simulink model "Distribution_v2"  (Simulink 7.9)
settings: Solver=VariableStepDiscrete  StartTime=0.0  StopTime=1000  RelTol=1e-3
libraries: simeventslib x35
(part 1 of 6)
settings Model: Creator=tsprock3  LastModifiedBy=tsprock3
settings DebuggingCC: SimStateOlderReleaseMsg=warning

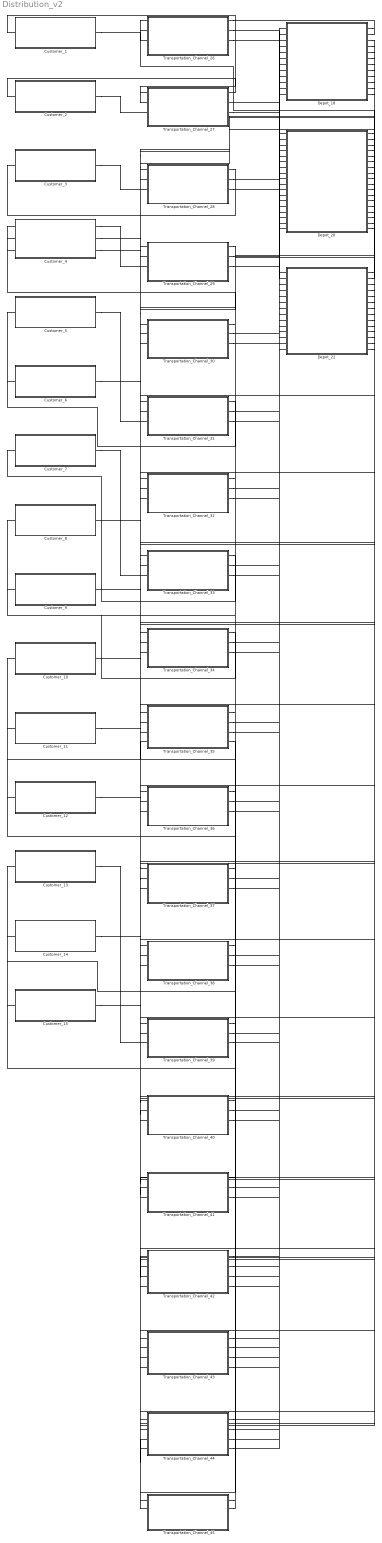
== system Distribution_v2 ==
  Customer_1 : Subsystem
  Customer_10 : Subsystem
  Customer_11 : Subsystem
  Customer_12 : Subsystem
  Customer_13 : Subsystem
  Customer_14 : Subsystem
  Customer_15 : Subsystem
  Customer_2 : Subsystem
  Customer_3 : Subsystem
  Customer_4 : Subsystem
  Customer_5 : Subsystem
  Customer_6 : Subsystem
  Customer_7 : Subsystem
  Customer_8 : Subsystem
  Customer_9 : Subsystem
  Depot_18 : Subsystem
  Depot_20 : Subsystem
  Depot_22 : Subsystem
  Transportation_Channel_26 : Subsystem
  Transportation_Channel_27 : Subsystem
  Transportation_Channel_28 : Subsystem
  Transportation_Channel_29 : Subsystem
  Transportation_Channel_30 : Subsystem
  Transportation_Channel_31 : Subsystem
  Transportation_Channel_32 : Subsystem
  Transportation_Channel_33 : Subsystem
  Transportation_Channel_34 : Subsystem
  Transportation_Channel_35 : Subsystem
  Transportation_Channel_36 : Subsystem
  Transportation_Channel_37 : Subsystem
  Transportation_Channel_38 : Subsystem
  Transportation_Channel_39 : Subsystem
  Transportation_Channel_40 : Subsystem
  Transportation_Channel_41 : Subsystem
  Transportation_Channel_42 : Subsystem
  Transportation_Channel_43 : Subsystem
  Transportation_Channel_44 : Subsystem
  Transportation_Channel_45 : Subsystem
  connections:
  Depot_22/RConn1 -- Transportation_Channel_26/LConn1
  Transportation_Channel_26/RConn1 -- Customer_1/LConn1
  Depot_22/RConn2 -- Transportation_Channel_26/LConn2
  Transportation_Channel_26/RConn2 -- Depot_22/LConn1
  Customer_1/RConn1 -- Transportation_Channel_26/LConn3
  Transportation_Channel_26/RConn3 -- Depot_22/LConn2
  Depot_18/RConn1 -- Transportation_Channel_27/LConn1
  Transportation_Channel_27/RConn1 -- Customer_2/LConn1
  Depot_18/RConn2 -- Transportation_Channel_27/LConn2
  Transportation_Channel_27/RConn2 -- Depot_18/LConn1
  Customer_2/RConn1 -- Transportation_Channel_27/LConn3
  Transportation_Channel_27/RConn3 -- Depot_18/LConn2
  Depot_20/RConn1 -- Transportation_Channel_28/LConn1
  Transportation_Channel_28/RConn1 -- Customer_3/LConn1
  Depot_20/RConn2 -- Transportation_Channel_28/LConn2
  Transportation_Channel_28/RConn2 -- Depot_20/LConn1
  Customer_3/RConn1 -- Transportation_Channel_28/LConn3
  Transportation_Channel_28/RConn3 -- Depot_20/LConn2
  Depot_18/RConn3 -- Transportation_Channel_29/LConn1
  Transportation_Channel_29/RConn1 -- Customer_4/LConn1
  Depot_18/RConn4 -- Transportation_Channel_29/LConn2
  Transportation_Channel_29/RConn2 -- Depot_18/LConn3
  Customer_4/RConn1 -- Transportation_Channel_29/LConn3
  Transportation_Channel_29/RConn3 -- Depot_18/LConn4
  Depot_20/RConn3 -- Transportation_Channel_30/LConn1
  Transportation_Channel_30/RConn1 -- Customer_4/LConn2
  Depot_20/RConn4 -- Transportation_Channel_30/LConn2
  Transportation_Channel_30/RConn2 -- Depot_20/LConn3
  Customer_4/RConn2 -- Transportation_Channel_30/LConn3
  Transportation_Channel_30/RConn3 -- Depot_20/LConn4
  Depot_22/RConn3 -- Transportation_Channel_31/LConn1
  Transportation_Channel_31/RConn1 -- Customer_5/LConn1
  Depot_22/RConn4 -- Transportation_Channel_31/LConn2
  Transportation_Channel_31/RConn2 -- Depot_22/LConn3
  Customer_5/RConn1 -- Transportation_Channel_31/LConn3
  Transportation_Channel_31/RConn3 -- Depot_22/LConn4
  Depot_18/RConn5 -- Transportation_Channel_32/LConn1
  Transportation_Channel_32/RConn1 -- Customer_6/LConn1
  Depot_18/RConn6 -- Transportation_Channel_32/LConn2
  Transportation_Channel_32/RConn2 -- Depot_18/LConn5
  Customer_6/RConn1 -- Transportation_Channel_32/LConn3
  Transportation_Channel_32/RConn3 -- Depot_18/LConn6
  Depot_20/RConn5 -- Transportation_Channel_33/LConn1
  Transportation_Channel_33/RConn1 -- Customer_7/LConn1
  Depot_20/RConn6 -- Transportation_Channel_33/LConn2
  Transportation_Channel_33/RConn2 -- Depot_20/LConn5
  Customer_7/RConn1 -- Transportation_Channel_33/LConn3
  Transportation_Channel_33/RConn3 -- Depot_20/LConn6
  Depot_20/RConn7 -- Transportation_Channel_34/LConn1
  Transportation_Channel_34/RConn1 -- Customer_8/LConn1
  Depot_20/RConn8 -- Transportation_Channel_34/LConn2
  Transportation_Channel_34/RConn2 -- Depot_20/LConn7
  Customer_8/RConn1 -- Transportation_Channel_34/LConn3
  Transportation_Channel_34/RConn3 -- Depot_20/LConn8
  Depot_18/RConn7 -- Transportation_Channel_35/LConn1
  Transportation_Channel_35/RConn1 -- Customer_9/LConn1
  Depot_18/RConn8 -- Transportation_Channel_35/LConn2
  Transportation_Channel_35/RConn2 -- Depot_18/LConn7
  Customer_9/RConn1 -- Transportation_Channel_35/LConn3
  Transportation_Channel_35/RConn3 -- Depot_18/LConn8
  Depot_22/RConn5 -- Transportation_Channel_36/LConn1
  Transportation_Channel_36/RConn1 -- Customer_10/LConn1
  Depot_22/RConn6 -- Transportation_Channel_36/LConn2
  Transportation_Channel_36/RConn2 -- Depot_22/LConn5
  Customer_10/RConn1 -- Transportation_Channel_36/LConn3
  Transportation_Channel_36/RConn3 -- Depot_22/LConn6
  Depot_20/RConn9 -- Transportation_Channel_37/LConn1
  Transportation_Channel_37/RConn1 -- Customer_11/LConn1
  Depot_20/RConn10 -- Transportation_Channel_37/LConn2
  Transportation_Channel_37/RConn2 -- Depot_20/LConn9
  Customer_11/RConn1 -- Transportation_Channel_37/LConn3
  Transportation_Channel_37/RConn3 -- Depot_20/LConn10
  Depot_22/RConn7 -- Transportation_Channel_38/LConn1
  Transportation_Channel_38/RConn1 -- Customer_12/LConn1
  Depot_22/RConn8 -- Transportation_Channel_38/LConn2
  Transportation_Channel_38/RConn2 -- Depot_22/LConn7
  Customer_12/RConn1 -- Transportation_Channel_38/LConn3
  Transportation_Channel_38/RConn3 -- Depot_22/LConn8
  Depot_22/RConn9 -- Transportation_Channel_39/LConn1
  Transportation_Channel_39/RConn1 -- Customer_13/LConn1
  Depot_22/RConn10 -- Transportation_Channel_39/LConn2
  Transportation_Channel_39/RConn2 -- Depot_22/LConn9
  Customer_13/RConn1 -- Transportation_Channel_39/LConn3
  Transportation_Channel_39/RConn3 -- Depot_22/LConn10
  Depot_20/RConn11 -- Transportation_Channel_40/LConn1
  Transportation_Channel_40/RConn1 -- Customer_14/LConn1
  Depot_20/RConn12 -- Transportation_Channel_40/LConn2
  Transportation_Channel_40/RConn2 -- Depot_20/LConn11
  Customer_14/RConn1 -- Transportation_Channel_40/LConn3
  Transportation_Channel_40/RConn3 -- Depot_20/LConn12
  Depot_20/RConn13 -- Transportation_Channel_41/LConn1
  Transportation_Channel_41/RConn1 -- Customer_15/LConn1
  Depot_20/RConn14 -- Transportation_Channel_41/LConn2
  Transportation_Channel_41/RConn2 -- Depot_20/LConn13
  Customer_15/RConn1 -- Transportation_Channel_41/LConn3
  Transportation_Channel_41/RConn3 -- Depot_20/LConn14
  Depot_20/RConn15 -- Transportation_Channel_42/LConn1
  Transportation_Channel_42/RConn1 -- Depot_18/LConn9
  Depot_20/RConn16 -- Transportation_Channel_42/LConn2
  Transportation_Channel_42/RConn2 -- Depot_20/LConn15
  Depot_18/RConn9 -- Transportation_Channel_42/LConn3
  Transportation_Channel_42/RConn3 -- Depot_20/LConn16
  Depot_18/RConn10 -- Transportation_Channel_42/LConn4
  Transportation_Channel_42/RConn4 -- Depot_18/LConn10
  Depot_22/RConn11 -- Transportation_Channel_43/LConn1
  Transportation_Channel_43/RConn1 -- Depot_18/LConn11
  Depot_22/RConn12 -- Transportation_Channel_43/LConn2
  Transportation_Channel_43/RConn2 -- Depot_22/LConn11
  Depot_18/RConn11 -- Transportation_Channel_43/LConn3
  Transportation_Channel_43/RConn3 -- Depot_22/LConn12
  Depot_18/RConn12 -- Transportation_Channel_43/LConn4
  Transportation_Channel_43/RConn4 -- Depot_18/LConn12
  Depot_22/RConn13 -- Transportation_Channel_44/LConn1
  Transportation_Channel_44/RConn1 -- Depot_20/LConn17
  Depot_22/RConn14 -- Transportation_Channel_44/LConn2
  Transportation_Channel_44/RConn2 -- Depot_22/LConn13
  Depot_20/RConn17 -- Transportation_Channel_44/LConn3
  Transportation_Channel_44/RConn3 -- Depot_22/LConn14
  Depot_20/RConn18 -- Transportation_Channel_44/LConn4
  Transportation_Channel_44/RConn4 -- Depot_20/LConn18
  Transportation_Channel_35/RConn4 -- Transportation_Channel_45/LConn1
  Transportation_Channel_45/RConn1 -- Customer_4/LConn3
  Customer_4/RConn3 -- Transportation_Channel_45/LConn2
  Transportation_Channel_45/RConn2 -- Transportation_Channel_35/LConn4

== system Distribution_v2/Customer_1 ==
  Commodity_1 : Subsystem  mask{Mean=2000/340, AttributeValue=[1  22  18   2]|1|2|1}
      mask prompts: Mean "Frequency"; AttributeValue "Attributes"
  Commodity_2 : Subsystem  mask{Mean=2000/60, AttributeValue=[1  22  18   4]|1|4|1}
      mask prompts: Mean "Frequency"; AttributeValue "Attributes"
  Commodity_3 : Subsystem  mask{Mean=2000/480, AttributeValue=[1  22   5   0]|1|5|1}
      mask prompts: Mean "Frequency"; AttributeValue "Attributes"
  Commodity_4 : Subsystem  mask{Mean=2000/293, AttributeValue=[1  22  18   6]|1|6|1}
      mask prompts: Mean "Frequency"; AttributeValue "Attributes"
  Commodity_5 : Subsystem  mask{Mean=2000/376, AttributeValue=[1  22  20   7]|1|7|1}
      mask prompts: Mean "Frequency"; AttributeValue "Attributes"
  Commodity_6 : Subsystem  mask{Mean=2000/253, AttributeValue=[1  22  20   8]|1|8|1}
      mask prompts: Mean "Frequency"; AttributeValue "Attributes"
  Commodity_7 : Subsystem  mask{Mean=2000/75, AttributeValue=[1  22  13   0]|1|13|1}
      mask prompts: Mean "Frequency"; AttributeValue "Attributes"
  Commodity_8 : Subsystem  mask{Mean=2000/421, AttributeValue=[1  22  20  14]|1|14|1}
      mask prompts: Mean "Frequency"; AttributeValue "Attributes"
  Commodity_9 : Subsystem  mask{Mean=2000/408, AttributeValue=[1  22  20  15]|1|15|1}
      mask prompts: Mean "Frequency"; AttributeValue "Attributes"
  Entity Sink : EntitySink
  Get Attribute : GetAttribute  AttributeName=Origin|Destination|Start  AttributeMissing=Error|Error|Error  AttributeDefaultValue=1|1|1  AttributeTreatAsVector=1|1|1  AttributeSendTiming=After entity departure|After entity departure|After entity departure  EvaluatedDefaultAttributeValue={[];[];[]}
      settings: OutputPortMap=o1,o2,o3
  Get Attribute1 : GetAttribute  AttributeName=Route  EvaluatedDefaultAttributeValue={[]}
      settings: OutputPortMap=o1
  IN_Commodity : PathCombiner  NumberInputPorts=9
  IN_Shipment : PathCombiner  NumberInputPorts=1
  Lookup : Constant  Value=[22]
  MATLAB Function : MATLAB Function  TreatAsAtomicUnit=on
  Mux : Mux  Inputs=3
  Node_ID : Constant
  OUT_Shipment : OutputSwitch  NumberOutputPorts=1  SwitchingCriterion=From signal port p  AttributeName=Customer
  Shipment_Metrics : simeventslib/SimEvents Sinks/Discrete Event Signal to Workspace  VariableName=Customer_1  SaveFormat=Structure With Time  isMonitorOnly=off  isRecordIC=off
  Single Server : SingleServer  ServiceTime=0
  Timed to Evnt Signal : TimedToEventSignal
  Timed to Evnt Signal1 : TimedToEventSignal
  IN_Shipment_1 : PMIOPort  Port=1  Side=Left
  OUT_Shipment_1 : PMIOPort  Port=2  Side=Right
  wires:
  Timed to Evnt Signal1/1 -> MATLAB Function/3(lookup)
  Lookup/1 -> Timed to Evnt Signal1/1
  Timed to Evnt Signal/1 -> MATLAB Function/2(current)
  Get Attribute1/1 -> MATLAB Function/1(route)
  MATLAB Function/1(next) -> OUT_Shipment/1
  Node_ID/1 -> Timed to Evnt Signal/1
  Mux/1 -> Shipment_Metrics/1
  Get Attribute/3 -> Mux/3
  Get Attribute/2 -> Mux/2
  Get Attribute/1 -> Mux/1
  connections:
  Single Server/RConn1 -- OUT_Shipment/LConn1
  Get Attribute1/RConn1 -- Single Server/LConn1
  IN_Commodity/RConn1 -- Get Attribute1/LConn1
  Get Attribute/LConn1 -- IN_Shipment/RConn1
  Entity Sink/LConn1 -- Get Attribute/RConn1
  IN_Shipment/LConn1 -- IN_Shipment_1/RConn1
  OUT_Shipment/RConn1 -- OUT_Shipment_1/RConn1
  Commodity_1/RConn1 -- IN_Commodity/LConn1
  Commodity_2/RConn1 -- IN_Commodity/LConn2
  Commodity_3/RConn1 -- IN_Commodity/LConn3
  Commodity_4/RConn1 -- IN_Commodity/LConn4
  Commodity_5/RConn1 -- IN_Commodity/LConn5
  Commodity_6/RConn1 -- IN_Commodity/LConn6
  Commodity_7/RConn1 -- IN_Commodity/LConn7
  Commodity_8/RConn1 -- IN_Commodity/LConn8
  Commodity_9/RConn1 -- IN_Commodity/LConn9

== system Distribution_v2/Customer_10 ==
  Commodity_75 : Subsystem  mask{Mean=2000/245, AttributeValue=[10  22  18   4]|10|4|1}
      mask prompts: Mean "Frequency"; AttributeValue "Attributes"
  Commodity_76 : Subsystem  mask{Mean=2000/184, AttributeValue=[10  22  20   7]|10|7|1}
      mask prompts: Mean "Frequency"; AttributeValue "Attributes"
  Commodity_77 : Subsystem  mask{Mean=2000/443, AttributeValue=[10  22  18   9]|10|9|1}
      mask prompts: Mean "Frequency"; AttributeValue "Attributes"
  Commodity_78 : Subsystem  mask{Mean=2000/131, AttributeValue=[10  22  13   0]|10|13|1}
      mask prompts: Mean "Frequency"; AttributeValue "Attributes"
  Commodity_79 : Subsystem  mask{Mean=2000/340, AttributeValue=[10  22  20  14]|10|14|1}
      mask prompts: Mean "Frequency"; AttributeValue "Attributes"
  Commodity_80 : Subsystem  mask{Mean=2000/361, AttributeValue=[10  22  20  15]|10|15|1}
      mask prompts: Mean "Frequency"; AttributeValue "Attributes"
  Entity Sink : EntitySink
  Get Attribute : GetAttribute  AttributeName=Origin|Destination|Start  AttributeMissing=Error|Error|Error  AttributeDefaultValue=1|1|1  AttributeTreatAsVector=1|1|1  AttributeSendTiming=After entity departure|After entity departure|After entity departure  EvaluatedDefaultAttributeValue={[];[];[]}
      settings: OutputPortMap=o1,o2,o3
  Get Attribute1 : GetAttribute  AttributeName=Route  EvaluatedDefaultAttributeValue={[]}
      settings: OutputPortMap=o1
  IN_Commodity : PathCombiner  NumberInputPorts=6
  IN_Shipment : PathCombiner  NumberInputPorts=1
  Lookup : Constant  Value=[22]
  MATLAB Function : MATLAB Function  TreatAsAtomicUnit=on
  Mux : Mux  Inputs=3
  Node_ID : Constant  Value=10
  OUT_Shipment : OutputSwitch  NumberOutputPorts=1  SwitchingCriterion=From signal port p  AttributeName=Customer
  Shipment_Metrics : simeventslib/SimEvents Sinks/Discrete Event Signal to Workspace  VariableName=Customer_10  SaveFormat=Structure With Time  isMonitorOnly=off  isRecordIC=off
  Single Server : SingleServer  ServiceTime=0
  Timed to Evnt Signal : TimedToEventSignal
  Timed to Evnt Signal1 : TimedToEventSignal
  IN_Shipment_1 : PMIOPort  Port=1  Side=Left
  OUT_Shipment_1 : PMIOPort  Port=2  Side=Right
  wires:
  Timed to Evnt Signal1/1 -> MATLAB Function/3(lookup)
  Lookup/1 -> Timed to Evnt Signal1/1
  Timed to Evnt Signal/1 -> MATLAB Function/2(current)
  Get Attribute1/1 -> MATLAB Function/1(route)
  MATLAB Function/1(next) -> OUT_Shipment/1
  Node_ID/1 -> Timed to Evnt Signal/1
  Mux/1 -> Shipment_Metrics/1
  Get Attribute/3 -> Mux/3
  Get Attribute/2 -> Mux/2
  Get Attribute/1 -> Mux/1
  connections:
  Single Server/RConn1 -- OUT_Shipment/LConn1
  Get Attribute1/RConn1 -- Single Server/LConn1
  IN_Commodity/RConn1 -- Get Attribute1/LConn1
  Get Attribute/LConn1 -- IN_Shipment/RConn1
  Entity Sink/LConn1 -- Get Attribute/RConn1
  IN_Shipment/LConn1 -- IN_Shipment_1/RConn1
  OUT_Shipment/RConn1 -- OUT_Shipment_1/RConn1
  Commodity_75/RConn1 -- IN_Commodity/LConn1
  Commodity_76/RConn1 -- IN_Commodity/LConn2
  Commodity_77/RConn1 -- IN_Commodity/LConn3
  Commodity_78/RConn1 -- IN_Commodity/LConn4
  Commodity_79/RConn1 -- IN_Commodity/LConn5
  Commodity_80/RConn1 -- IN_Commodity/LConn6

== system Distribution_v2/Customer_11 ==
  Commodity_81 : Subsystem  mask{Mean=2000/327, AttributeValue=[11  20  22   1]|11|1|1}
      mask prompts: Mean "Frequency"; AttributeValue "Attributes"
  Commodity_82 : Subsystem  mask{Mean=2000/390, AttributeValue=[11  20  18   2]|11|2|1}
      mask prompts: Mean "Frequency"; AttributeValue "Attributes"
  Commodity_83 : Subsystem  mask{Mean=2000/350, AttributeValue=[11  20  18   6]|11|6|1}
      mask prompts: Mean "Frequency"; AttributeValue "Attributes"
  Commodity_84 : Subsystem  mask{Mean=2000/16, AttributeValue=[11  20   7   0]|11|7|1}
      mask prompts: Mean "Frequency"; AttributeValue "Attributes"
  Commodity_85 : Subsystem  mask{Mean=2000/453, AttributeValue=[11  20  22  10]|11|10|1}
      mask prompts: Mean "Frequency"; AttributeValue "Attributes"
  Entity Sink : EntitySink
  Get Attribute : GetAttribute  AttributeName=Origin|Destination|Start  AttributeMissing=Error|Error|Error  AttributeDefaultValue=1|1|1  AttributeTreatAsVector=1|1|1  AttributeSendTiming=After entity departure|After entity departure|After entity departure  EvaluatedDefaultAttributeValue={[];[];[]}
      settings: OutputPortMap=o1,o2,o3
  Get Attribute1 : GetAttribute  AttributeName=Route  EvaluatedDefaultAttributeValue={[]}
      settings: OutputPortMap=o1
  IN_Commodity : PathCombiner  NumberInputPorts=5
  IN_Shipment : PathCombiner  NumberInputPorts=1
  Lookup : Constant  Value=[20]
  MATLAB Function : MATLAB Function  TreatAsAtomicUnit=on
  Mux : Mux  Inputs=3
  Node_ID : Constant  Value=11
  OUT_Shipment : OutputSwitch  NumberOutputPorts=1  SwitchingCriterion=From signal port p  AttributeName=Customer
  Shipment_Metrics : simeventslib/SimEvents Sinks/Discrete Event Signal to Workspace  VariableName=Customer_11  SaveFormat=Structure With Time  isMonitorOnly=off  isRecordIC=off
  Single Server : SingleServer  ServiceTime=0
  Timed to Evnt Signal : TimedToEventSignal
  Timed to Evnt Signal1 : TimedToEventSignal
  IN_Shipment_1 : PMIOPort  Port=1  Side=Left
  OUT_Shipment_1 : PMIOPort  Port=2  Side=Right
  wires:
  Timed to Evnt Signal1/1 -> MATLAB Function/3(lookup)
  Lookup/1 -> Timed to Evnt Signal1/1
  Timed to Evnt Signal/1 -> MATLAB Function/2(current)
  Get Attribute1/1 -> MATLAB Function/1(route)
  MATLAB Function/1(next) -> OUT_Shipment/1
  Node_ID/1 -> Timed to Evnt Signal/1
  Mux/1 -> Shipment_Metrics/1
  Get Attribute/3 -> Mux/3
  Get Attribute/2 -> Mux/2
  Get Attribute/1 -> Mux/1
  connections:
  Single Server/RConn1 -- OUT_Shipment/LConn1
  Get Attribute1/RConn1 -- Single Server/LConn1
  IN_Commodity/RConn1 -- Get Attribute1/LConn1
  Get Attribute/LConn1 -- IN_Shipment/RConn1
  Entity Sink/LConn1 -- Get Attribute/RConn1
  IN_Shipment/LConn1 -- IN_Shipment_1/RConn1
  OUT_Shipment/RConn1 -- OUT_Shipment_1/RConn1
  Commodity_81/RConn1 -- IN_Commodity/LConn1
  Commodity_82/RConn1 -- IN_Commodity/LConn2
  Commodity_83/RConn1 -- IN_Commodity/LConn3
  Commodity_84/RConn1 -- IN_Commodity/LConn4
  Commodity_85/RConn1 -- IN_Commodity/LConn5

== system Distribution_v2/Customer_12 ==
  Commodity_86 : Subsystem  mask{Mean=2000/120, AttributeValue=[12  22  18   2]|12|2|1}
      mask prompts: Mean "Frequency"; AttributeValue "Attributes"
  Commodity_87 : Subsystem  mask{Mean=2000/245, AttributeValue=[12  22  18   4]|12|4|1}
      mask prompts: Mean "Frequency"; AttributeValue "Attributes"
  Commodity_88 : Subsystem  mask{Mean=2000/490, AttributeValue=[12  22   5   0]|12|5|1}
      mask prompts: Mean "Frequency"; AttributeValue "Attributes"
  Commodity_89 : Subsystem  mask{Mean=2000/30, AttributeValue=[12  22  20   8]|12|8|1}
      mask prompts: Mean "Frequency"; AttributeValue "Attributes"
  Commodity_90 : Subsystem  mask{Mean=2000/36, AttributeValue=[12  22  10   0]|12|10|1}
      mask prompts: Mean "Frequency"; AttributeValue "Attributes"
  Commodity_91 : Subsystem  mask{Mean=2000/410, AttributeValue=[12  22  13   0]|12|13|1}
      mask prompts: Mean "Frequency"; AttributeValue "Attributes"
  Entity Sink : EntitySink
  Get Attribute : GetAttribute  AttributeName=Origin|Destination|Start  AttributeMissing=Error|Error|Error  AttributeDefaultValue=1|1|1  AttributeTreatAsVector=1|1|1  AttributeSendTiming=After entity departure|After entity departure|After entity departure  EvaluatedDefaultAttributeValue={[];[];[]}
      settings: OutputPortMap=o1,o2,o3
  Get Attribute1 : GetAttribute  AttributeName=Route  EvaluatedDefaultAttributeValue={[]}
      settings: OutputPortMap=o1
  IN_Commodity : PathCombiner  NumberInputPorts=6
  IN_Shipment : PathCombiner  NumberInputPorts=1
  Lookup : Constant  Value=[22]
  MATLAB Function : MATLAB Function  TreatAsAtomicUnit=on
  Mux : Mux  Inputs=3
  Node_ID : Constant  Value=12
  OUT_Shipment : OutputSwitch  NumberOutputPorts=1  SwitchingCriterion=From signal port p  AttributeName=Customer
  Shipment_Metrics : simeventslib/SimEvents Sinks/Discrete Event Signal to Workspace  VariableName=Customer_12  SaveFormat=Structure With Time  isMonitorOnly=off  isRecordIC=off
  Single Server : SingleServer  ServiceTime=0
  Timed to Evnt Signal : TimedToEventSignal
  Timed to Evnt Signal1 : TimedToEventSignal
  IN_Shipment_1 : PMIOPort  Port=1  Side=Left
  OUT_Shipment_1 : PMIOPort  Port=2  Side=Right
  wires:
  Timed to Evnt Signal1/1 -> MATLAB Function/3(lookup)
  Lookup/1 -> Timed to Evnt Signal1/1
  Timed to Evnt Signal/1 -> MATLAB Function/2(current)
  Get Attribute1/1 -> MATLAB Function/1(route)
  MATLAB Function/1(next) -> OUT_Shipment/1
  Node_ID/1 -> Timed to Evnt Signal/1
  Mux/1 -> Shipment_Metrics/1
  Get Attribute/3 -> Mux/3
  Get Attribute/2 -> Mux/2
  Get Attribute/1 -> Mux/1
  connections:
  Single Server/RConn1 -- OUT_Shipment/LConn1
  Get Attribute1/RConn1 -- Single Server/LConn1
  IN_Commodity/RConn1 -- Get Attribute1/LConn1
  Get Attribute/LConn1 -- IN_Shipment/RConn1
  Entity Sink/LConn1 -- Get Attribute/RConn1
  IN_Shipment/LConn1 -- IN_Shipment_1/RConn1
  OUT_Shipment/RConn1 -- OUT_Shipment_1/RConn1
  Commodity_86/RConn1 -- IN_Commodity/LConn1
  Commodity_87/RConn1 -- IN_Commodity/LConn2
  Commodity_88/RConn1 -- IN_Commodity/LConn3
  Commodity_89/RConn1 -- IN_Commodity/LConn4
  Commodity_90/RConn1 -- IN_Commodity/LConn5
  Commodity_91/RConn1 -- IN_Commodity/LConn6

== system Distribution_v2/Customer_13 ==
  Commodity_92 : Subsystem  mask{Mean=2000/330, AttributeValue=[13  22   1   0]|13|1|1}
      mask prompts: Mean "Frequency"; AttributeValue "Attributes"
  Commodity_93 : Subsystem  mask{Mean=2000/217, AttributeValue=[13  22  18   6]|13|6|1}
      mask prompts: Mean "Frequency"; AttributeValue "Attributes"
  Commodity_94 : Subsystem  mask{Mean=2000/67, AttributeValue=[13  22  20   8]|13|8|1}
      mask prompts: Mean "Frequency"; AttributeValue "Attributes"
  Commodity_95 : Subsystem  mask{Mean=2000/196, AttributeValue=[13  22  18   9]|13|9|1}
      mask prompts: Mean "Frequency"; AttributeValue "Attributes"
  Commodity_96 : Subsystem  mask{Mean=2000/200, AttributeValue=[13  22  12   0]|13|12|1}
      mask prompts: Mean "Frequency"; AttributeValue "Attributes"
  Commodity_97 : Subsystem  mask{Mean=2000/329, AttributeValue=[13  22  20  15]|13|15|1}
      mask prompts: Mean "Frequency"; AttributeValue "Attributes"
  Entity Sink : EntitySink
  Get Attribute : GetAttribute  AttributeName=Origin|Destination|Start  AttributeMissing=Error|Error|Error  AttributeDefaultValue=1|1|1  AttributeTreatAsVector=1|1|1  AttributeSendTiming=After entity departure|After entity departure|After entity departure  EvaluatedDefaultAttributeValue={[];[];[]}
      settings: OutputPortMap=o1,o2,o3
  Get Attribute1 : GetAttribute  AttributeName=Route  EvaluatedDefaultAttributeValue={[]}
      settings: OutputPortMap=o1
  IN_Commodity : PathCombiner  NumberInputPorts=6
  IN_Shipment : PathCombiner  NumberInputPorts=1
  Lookup : Constant  Value=[22]
  MATLAB Function : MATLAB Function  TreatAsAtomicUnit=on
  Mux : Mux  Inputs=3
  Node_ID : Constant  Value=13
  OUT_Shipment : OutputSwitch  NumberOutputPorts=1  SwitchingCriterion=From signal port p  AttributeName=Customer
  Shipment_Metrics : simeventslib/SimEvents Sinks/Discrete Event Signal to Workspace  VariableName=Customer_13  SaveFormat=Structure With Time  isMonitorOnly=off  isRecordIC=off
  Single Server : SingleServer  ServiceTime=0
  Timed to Evnt Signal : TimedToEventSignal
  Timed to Evnt Signal1 : TimedToEventSignal
  IN_Shipment_1 : PMIOPort  Port=1  Side=Left
  OUT_Shipment_1 : PMIOPort  Port=2  Side=Right
  wires:
  Timed to Evnt Signal1/1 -> MATLAB Function/3(lookup)
  Lookup/1 -> Timed to Evnt Signal1/1
  Timed to Evnt Signal/1 -> MATLAB Function/2(current)
  Get Attribute1/1 -> MATLAB Function/1(route)
  MATLAB Function/1(next) -> OUT_Shipment/1
  Node_ID/1 -> Timed to Evnt Signal/1
  Mux/1 -> Shipment_Metrics/1
  Get Attribute/3 -> Mux/3
  Get Attribute/2 -> Mux/2
  Get Attribute/1 -> Mux/1
  connections:
  Single Server/RConn1 -- OUT_Shipment/LConn1
  Get Attribute1/RConn1 -- Single Server/LConn1
  IN_Commodity/RConn1 -- Get Attribute1/LConn1
  Get Attribute/LConn1 -- IN_Shipment/RConn1
  Entity Sink/LConn1 -- Get Attribute/RConn1
  IN_Shipment/LConn1 -- IN_Shipment_1/RConn1
  OUT_Shipment/RConn1 -- OUT_Shipment_1/RConn1
  Commodity_92/RConn1 -- IN_Commodity/LConn1
  Commodity_93/RConn1 -- IN_Commodity/LConn2
  Commodity_94/RConn1 -- IN_Commodity/LConn3
  Commodity_95/RConn1 -- IN_Commodity/LConn4
  Commodity_96/RConn1 -- IN_Commodity/LConn5
  Commodity_97/RConn1 -- IN_Commodity/LConn6

== system Distribution_v2/Customer_14 ==
  Commodity_100 : Subsystem  mask{Mean=2000/54, AttributeValue=[14  20  18   4]|14|4|1}
      mask prompts: Mean "Frequency"; AttributeValue "Attributes"
  Commodity_101 : Subsystem  mask{Mean=2000/100, AttributeValue=[14  20  22   5]|14|5|1}
      mask prompts: Mean "Frequency"; AttributeValue "Attributes"
  Commodity_102 : Subsystem  mask{Mean=2000/170, AttributeValue=[14  20  18   6]|14|6|1}
      mask prompts: Mean "Frequency"; AttributeValue "Attributes"
  Commodity_103 : Subsystem  mask{Mean=2000/369, AttributeValue=[14  20  18   9]|14|9|1}
      mask prompts: Mean "Frequency"; AttributeValue "Attributes"
  Commodity_104 : Subsystem  mask{Mean=2000/212, AttributeValue=[14  20  22  10]|14|10|1}
      mask prompts: Mean "Frequency"; AttributeValue "Attributes"
  Commodity_105 : Subsystem  mask{Mean=2000/492, AttributeValue=[14  20  22  13]|14|13|1}
      mask prompts: Mean "Frequency"; AttributeValue "Attributes"
  Commodity_106 : Subsystem  mask{Mean=2000/351, AttributeValue=[14  20  15   0]|14|15|1}
      mask prompts: Mean "Frequency"; AttributeValue "Attributes"
  Commodity_98 : Subsystem  mask{Mean=2000/216, AttributeValue=[14  20  18   2]|14|2|1}
      mask prompts: Mean "Frequency"; AttributeValue "Attributes"
  Commodity_99 : Subsystem  mask{Mean=2000/493, AttributeValue=[14  20   3   0]|14|3|1}
      mask prompts: Mean "Frequency"; AttributeValue "Attributes"
  Entity Sink : EntitySink
  Get Attribute : GetAttribute  AttributeName=Origin|Destination|Start  AttributeMissing=Error|Error|Error  AttributeDefaultValue=1|1|1  AttributeTreatAsVector=1|1|1  AttributeSendTiming=After entity departure|After entity departure|After entity departure  EvaluatedDefaultAttributeValue={[];[];[]}
      settings: OutputPortMap=o1,o2,o3
  Get Attribute1 : GetAttribute  AttributeName=Route  EvaluatedDefaultAttributeValue={[]}
      settings: OutputPortMap=o1
  IN_Commodity : PathCombiner  NumberInputPorts=9
  IN_Shipment : PathCombiner  NumberInputPorts=1
  Lookup : Constant  Value=[20]
  MATLAB Function : MATLAB Function  TreatAsAtomicUnit=on
  Mux : Mux  Inputs=3
  Node_ID : Constant  Value=14
  OUT_Shipment : OutputSwitch  NumberOutputPorts=1  SwitchingCriterion=From signal port p  AttributeName=Customer
  Shipment_Metrics : simeventslib/SimEvents Sinks/Discrete Event Signal to Workspace  VariableName=Customer_14  SaveFormat=Structure With Time  isMonitorOnly=off  isRecordIC=off
  Single Server : SingleServer  ServiceTime=0
  Timed to Evnt Signal : TimedToEventSignal
  Timed to Evnt Signal1 : TimedToEventSignal
  IN_Shipment_1 : PMIOPort  Port=1  Side=Left
  OUT_Shipment_1 : PMIOPort  Port=2  Side=Right
  wires:
  Timed to Evnt Signal1/1 -> MATLAB Function/3(lookup)
  Lookup/1 -> Timed to Evnt Signal1/1
  Timed to Evnt Signal/1 -> MATLAB Function/2(current)
  Get Attribute1/1 -> MATLAB Function/1(route)
  MATLAB Function/1(next) -> OUT_Shipment/1
  Node_ID/1 -> Timed to Evnt Signal/1
  Mux/1 -> Shipment_Metrics/1
  Get Attribute/3 -> Mux/3
  Get Attribute/2 -> Mux/2
  Get Attribute/1 -> Mux/1
  connections:
  Single Server/RConn1 -- OUT_Shipment/LConn1
  Get Attribute1/RConn1 -- Single Server/LConn1
  IN_Commodity/RConn1 -- Get Attribute1/LConn1
  Get Attribute/LConn1 -- IN_Shipment/RConn1
  Entity Sink/LConn1 -- Get Attribute/RConn1
  IN_Shipment/LConn1 -- IN_Shipment_1/RConn1
  OUT_Shipment/RConn1 -- OUT_Shipment_1/RConn1
  Commodity_98/RConn1 -- IN_Commodity/LConn1
  Commodity_99/RConn1 -- IN_Commodity/LConn2
  Commodity_100/RConn1 -- IN_Commodity/LConn3
  Commodity_101/RConn1 -- IN_Commodity/LConn4
  Commodity_102/RConn1 -- IN_Commodity/LConn5
  Commodity_103/RConn1 -- IN_Commodity/LConn6
  Commodity_104/RConn1 -- IN_Commodity/LConn7
  Commodity_105/RConn1 -- IN_Commodity/LConn8
  Commodity_106/RConn1 -- IN_Commodity/LConn9

== system Distribution_v2/Customer_15 ==
  Commodity_107 : Subsystem  mask{Mean=2000/65, AttributeValue=[15  20  22   5]|15|5|1}
      mask prompts: Mean "Frequency"; AttributeValue "Attributes"
  Commodity_108 : Subsystem  mask{Mean=2000/17, AttributeValue=[15  20   7   0]|15|7|1}
      mask prompts: Mean "Frequency"; AttributeValue "Attributes"
  Commodity_109 : Subsystem  mask{Mean=2000/185, AttributeValue=[15  20  11   0]|15|11|1}
      mask prompts: Mean "Frequency"; AttributeValue "Attributes"
  Commodity_110 : Subsystem  mask{Mean=2000/491, AttributeValue=[15  20  22  12]|15|12|1}
      mask prompts: Mean "Frequency"; AttributeValue "Attributes"
  Commodity_111 : Subsystem  mask{Mean=2000/428, AttributeValue=[15  20  22  13]|15|13|1}
      mask prompts: Mean "Frequency"; AttributeValue "Attributes"
  Entity Sink : EntitySink
  Get Attribute : GetAttribute  AttributeName=Origin|Destination|Start  AttributeMissing=Error|Error|Error  AttributeDefaultValue=1|1|1  AttributeTreatAsVector=1|1|1  AttributeSendTiming=After entity departure|After entity departure|After entity departure  EvaluatedDefaultAttributeValue={[];[];[]}
      settings: OutputPortMap=o1,o2,o3
  Get Attribute1 : GetAttribute  AttributeName=Route  EvaluatedDefaultAttributeValue={[]}
      settings: OutputPortMap=o1
  IN_Commodity : PathCombiner  NumberInputPorts=5
  IN_Shipment : PathCombiner  NumberInputPorts=1
  Lookup : Constant  Value=[20]
  MATLAB Function : MATLAB Function  TreatAsAtomicUnit=on
  Mux : Mux  Inputs=3
  Node_ID : Constant  Value=15
  OUT_Shipment : OutputSwitch  NumberOutputPorts=1  SwitchingCriterion=From signal port p  AttributeName=Customer
  Shipment_Metrics : simeventslib/SimEvents Sinks/Discrete Event Signal to Workspace  VariableName=Customer_15  SaveFormat=Structure With Time  isMonitorOnly=off  isRecordIC=off
  Single Server : SingleServer  ServiceTime=0
  Timed to Evnt Signal : TimedToEventSignal
  Timed to Evnt Signal1 : TimedToEventSignal
  IN_Shipment_1 : PMIOPort  Port=1  Side=Left
  OUT_Shipment_1 : PMIOPort  Port=2  Side=Right
  wires:
  Timed to Evnt Signal1/1 -> MATLAB Function/3(lookup)
  Lookup/1 -> Timed to Evnt Signal1/1
  Timed to Evnt Signal/1 -> MATLAB Function/2(current)
  Get Attribute1/1 -> MATLAB Function/1(route)
  MATLAB Function/1(next) -> OUT_Shipment/1
  Node_ID/1 -> Timed to Evnt Signal/1
  Mux/1 -> Shipment_Metrics/1
  Get Attribute/3 -> Mux/3
  Get Attribute/2 -> Mux/2
  Get Attribute/1 -> Mux/1
  connections:
  Single Server/RConn1 -- OUT_Shipment/LConn1
  Get Attribute1/RConn1 -- Single Server/LConn1
  IN_Commodity/RConn1 -- Get Attribute1/LConn1
  Get Attribute/LConn1 -- IN_Shipment/RConn1
  Entity Sink/LConn1 -- Get Attribute/RConn1
  IN_Shipment/LConn1 -- IN_Shipment_1/RConn1
  OUT_Shipment/RConn1 -- OUT_Shipment_1/RConn1
  Commodity_107/RConn1 -- IN_Commodity/LConn1
  Commodity_108/RConn1 -- IN_Commodity/LConn2
  Commodity_109/RConn1 -- IN_Commodity/LConn3
  Commodity_110/RConn1 -- IN_Commodity/LConn4
  Commodity_111/RConn1 -- IN_Commodity/LConn5

== system Distribution_v2/Customer_2 ==
  Commodity_10 : Subsystem  mask{Mean=2000/465, AttributeValue=[2  18  22   1]|2|1|1}
      mask prompts: Mean "Frequency"; AttributeValue "Attributes"
  Commodity_11 : Subsystem  mask{Mean=2000/99, AttributeValue=[2  18  20   3]|2|3|1}
      mask prompts: Mean "Frequency"; AttributeValue "Attributes"
  Commodity_12 : Subsystem  mask{Mean=2000/309, AttributeValue=[2  18   4   0]|2|4|1}
      mask prompts: Mean "Frequency"; AttributeValue "Attributes"
  Commodity_13 : Subsystem  mask{Mean=2000/176, AttributeValue=[2  18  22   5]|2|5|1}
      mask prompts: Mean "Frequency"; AttributeValue "Attributes"
  Commodity_14 : Subsystem  mask{Mean=2000/379, AttributeValue=[2  18  22  10]|2|10|1}
      mask prompts: Mean "Frequency"; AttributeValue "Attributes"
  Commodity_15 : Subsystem  mask{Mean=2000/284, AttributeValue=[2  18  22  12]|2|12|1}
      mask prompts: Mean "Frequency"; AttributeValue "Attributes"
  Commodity_16 : Subsystem  mask{Mean=2000/27, AttributeValue=[2  18  22  13]|2|13|1}
      mask prompts: Mean "Frequency"; AttributeValue "Attributes"
  Entity Sink : EntitySink
  Get Attribute : GetAttribute  AttributeName=Origin|Destination|Start  AttributeMissing=Error|Error|Error  AttributeDefaultValue=1|1|1  AttributeTreatAsVector=1|1|1  AttributeSendTiming=After entity departure|After entity departure|After entity departure  EvaluatedDefaultAttributeValue={[];[];[]}
      settings: OutputPortMap=o1,o2,o3
  Get Attribute1 : GetAttribute  AttributeName=Route  EvaluatedDefaultAttributeValue={[]}
      settings: OutputPortMap=o1
  IN_Commodity : PathCombiner  NumberInputPorts=7
  IN_Shipment : PathCombiner  NumberInputPorts=1
  Lookup : Constant  Value=[18]
  MATLAB Function : MATLAB Function  TreatAsAtomicUnit=on
  Mux : Mux  Inputs=3
  Node_ID : Constant  Value=2
  OUT_Shipment : OutputSwitch  NumberOutputPorts=1  SwitchingCriterion=From signal port p  AttributeName=Customer
  Shipment_Metrics : simeventslib/SimEvents Sinks/Discrete Event Signal to Workspace  VariableName=Customer_2  SaveFormat=Structure With Time  isMonitorOnly=off  isRecordIC=off
  Single Server : SingleServer  ServiceTime=0
  Timed to Evnt Signal : TimedToEventSignal
  Timed to Evnt Signal1 : TimedToEventSignal
  IN_Shipment_1 : PMIOPort  Port=1  Side=Left
  OUT_Shipment_1 : PMIOPort  Port=2  Side=Right
  wires:
  Timed to Evnt Signal1/1 -> MATLAB Function/3(lookup)
  Lookup/1 -> Timed to Evnt Signal1/1
  Timed to Evnt Signal/1 -> MATLAB Function/2(current)
  Get Attribute1/1 -> MATLAB Function/1(route)
  MATLAB Function/1(next) -> OUT_Shipment/1
  Node_ID/1 -> Timed to Evnt Signal/1
  Mux/1 -> Shipment_Metrics/1
  Get Attribute/3 -> Mux/3
  Get Attribute/2 -> Mux/2
  Get Attribute/1 -> Mux/1
  connections:
  Single Server/RConn1 -- OUT_Shipment/LConn1
  Get Attribute1/RConn1 -- Single Server/LConn1
  IN_Commodity/RConn1 -- Get Attribute1/LConn1
  Get Attribute/LConn1 -- IN_Shipment/RConn1
  Entity Sink/LConn1 -- Get Attribute/RConn1
  IN_Shipment/LConn1 -- IN_Shipment_1/RConn1
  OUT_Shipment/RConn1 -- OUT_Shipment_1/RConn1
  Commodity_10/RConn1 -- IN_Commodity/LConn1
  Commodity_11/RConn1 -- IN_Commodity/LConn2
  Commodity_12/RConn1 -- IN_Commodity/LConn3
  Commodity_13/RConn1 -- IN_Commodity/LConn4
  Commodity_14/RConn1 -- IN_Commodity/LConn5
  Commodity_15/RConn1 -- IN_Commodity/LConn6
  Commodity_16/RConn1 -- IN_Commodity/LConn7

== system Distribution_v2/Customer_3 ==
  Commodity_17 : Subsystem  mask{Mean=2000/285, AttributeValue=[3  20  18   2]|3|2|1}
      mask prompts: Mean "Frequency"; AttributeValue "Attributes"
  Commodity_18 : Subsystem  mask{Mean=2000/6, AttributeValue=[3  20  18   4]|3|4|1}
      mask prompts: Mean "Frequency"; AttributeValue "Attributes"
  Commodity_19 : Subsystem  mask{Mean=2000/82, AttributeValue=[3  20  22   5]|3|5|1}
      mask prompts: Mean "Frequency"; AttributeValue "Attributes"
  Commodity_20 : Subsystem  mask{Mean=2000/265, AttributeValue=[3  20   7   0]|3|7|1}
      mask prompts: Mean "Frequency"; AttributeValue "Attributes"
  Commodity_21 : Subsystem  mask{Mean=2000/301, AttributeValue=[3  20   8   0]|3|8|1}
      mask prompts: Mean "Frequency"; AttributeValue "Attributes"
  Commodity_22 : Subsystem  mask{Mean=2000/328, AttributeValue=[3  20  18   9]|3|9|1}
      mask prompts: Mean "Frequency"; AttributeValue "Attributes"
  Commodity_23 : Subsystem  mask{Mean=2000/42, AttributeValue=[3  20  22  12]|3|12|1}
      mask prompts: Mean "Frequency"; AttributeValue "Attributes"
  Commodity_24 : Subsystem  mask{Mean=2000/457, AttributeValue=[3  20  22  13]|3|13|1}
      mask prompts: Mean "Frequency"; AttributeValue "Attributes"
  Commodity_25 : Subsystem  mask{Mean=2000/413, AttributeValue=[3  20  14   0]|3|14|1}
      mask prompts: Mean "Frequency"; AttributeValue "Attributes"
  Entity Sink : EntitySink
  Get Attribute : GetAttribute  AttributeName=Origin|Destination|Start  AttributeMissing=Error|Error|Error  AttributeDefaultValue=1|1|1  AttributeTreatAsVector=1|1|1  AttributeSendTiming=After entity departure|After entity departure|After entity departure  EvaluatedDefaultAttributeValue={[];[];[]}
      settings: OutputPortMap=o1,o2,o3
  Get Attribute1 : GetAttribute  AttributeName=Route  EvaluatedDefaultAttributeValue={[]}
      settings: OutputPortMap=o1
  IN_Commodity : PathCombiner  NumberInputPorts=9
  IN_Shipment : PathCombiner  NumberInputPorts=1
  Lookup : Constant  Value=[20]
  MATLAB Function : MATLAB Function  TreatAsAtomicUnit=on
  Mux : Mux  Inputs=3
  Node_ID : Constant  Value=3
  OUT_Shipment : OutputSwitch  NumberOutputPorts=1  SwitchingCriterion=From signal port p  AttributeName=Customer
  Shipment_Metrics : simeventslib/SimEvents Sinks/Discrete Event Signal to Workspace  VariableName=Customer_3  SaveFormat=Structure With Time  isMonitorOnly=off  isRecordIC=off
  Single Server : SingleServer  ServiceTime=0
  Timed to Evnt Signal : TimedToEventSignal
  Timed to Evnt Signal1 : TimedToEventSignal
  IN_Shipment_1 : PMIOPort  Port=1  Side=Left
  OUT_Shipment_1 : PMIOPort  Port=2  Side=Right
  wires:
  Timed to Evnt Signal1/1 -> MATLAB Function/3(lookup)
  Lookup/1 -> Timed to Evnt Signal1/1
  Timed to Evnt Signal/1 -> MATLAB Function/2(current)
  Get Attribute1/1 -> MATLAB Function/1(route)
  MATLAB Function/1(next) -> OUT_Shipment/1
  Node_ID/1 -> Timed to Evnt Signal/1
  Mux/1 -> Shipment_Metrics/1
  Get Attribute/3 -> Mux/3
  Get Attribute/2 -> Mux/2
  Get Attribute/1 -> Mux/1
  connections:
  Single Server/RConn1 -- OUT_Shipment/LConn1
  Get Attribute1/RConn1 -- Single Server/LConn1
  IN_Commodity/RConn1 -- Get Attribute1/LConn1
  Get Attribute/LConn1 -- IN_Shipment/RConn1
  Entity Sink/LConn1 -- Get Attribute/RConn1
  IN_Shipment/LConn1 -- IN_Shipment_1/RConn1
  OUT_Shipment/RConn1 -- OUT_Shipment_1/RConn1
  Commodity_17/RConn1 -- IN_Commodity/LConn1
  Commodity_18/RConn1 -- IN_Commodity/LConn2
  Commodity_19/RConn1 -- IN_Commodity/LConn3
  Commodity_20/RConn1 -- IN_Commodity/LConn4
  Commodity_21/RConn1 -- IN_Commodity/LConn5
  Commodity_22/RConn1 -- IN_Commodity/LConn6
  Commodity_23/RConn1 -- IN_Commodity/LConn7
  Commodity_24/RConn1 -- IN_Commodity/LConn8
  Commodity_25/RConn1 -- IN_Commodity/LConn9

== system Distribution_v2/Customer_4 ==
  Commodity_26 : Subsystem  mask{Mean=2000/222, AttributeValue=[4  18   2   0]|4|2|1}
      mask prompts: Mean "Frequency"; AttributeValue "Attributes"
  Commodity_27 : Subsystem  mask{Mean=2000/481, AttributeValue=[4  18  20   3]|4|3|1}
      mask prompts: Mean "Frequency"; AttributeValue "Attributes"
  Commodity_28 : Subsystem  mask{Mean=2000/388, AttributeValue=[4  18  22   5]|4|5|1}
      mask prompts: Mean "Frequency"; AttributeValue "Attributes"
  Commodity_29 : Subsystem  mask{Mean=2000/200, AttributeValue=[4  18  20   8]|4|8|1}
      mask prompts: Mean "Frequency"; AttributeValue "Attributes"
  Commodity_30 : Subsystem  mask{Mean=2000/401, AttributeValue=[4  18   9   0]|4|9|1}
      mask prompts: Mean "Frequency"; AttributeValue "Attributes"
  Commodity_31 : Subsystem  mask{Mean=2000/456, AttributeValue=[4  18  22  10]|4|10|1}
      mask prompts: Mean "Frequency"; AttributeValue "Attributes"
  Commodity_32 : Subsystem  mask{Mean=2000/132, AttributeValue=[4  18  20  11]|4|11|1}
      mask prompts: Mean "Frequency"; AttributeValue "Attributes"
  Commodity_33 : Subsystem  mask{Mean=2000/69, AttributeValue=[4  18  22  12]|4|12|1}
      mask prompts: Mean "Frequency"; AttributeValue "Attributes"
  Entity Sink : EntitySink
  Get Attribute : GetAttribute  AttributeName=Origin|Destination|Start  AttributeMissing=Error|Error|Error  AttributeDefaultValue=1|1|1  AttributeTreatAsVector=1|1|1  AttributeSendTiming=After entity departure|After entity departure|After entity departure  EvaluatedDefaultAttributeValue={[];[];[]}
      settings: OutputPortMap=o1,o2,o3
  Get Attribute1 : GetAttribute  AttributeName=Route  EvaluatedDefaultAttributeValue={[]}
      settings: OutputPortMap=o1
  IN_Commodity : PathCombiner  NumberInputPorts=8
  IN_Shipment : PathCombiner
  Lookup : Constant  Value=[18,20,35]
  MATLAB Function : MATLAB Function  TreatAsAtomicUnit=on
  Mux : Mux  Inputs=3
  Node_ID : Constant  Value=4
  OUT_Shipment : OutputSwitch  SwitchingCriterion=From signal port p  AttributeName=Customer
  Shipment_Metrics : simeventslib/SimEvents Sinks/Discrete Event Signal to Workspace  VariableName=Customer_4  SaveFormat=Structure With Time  isMonitorOnly=off  isRecordIC=off
  Single Server : SingleServer  ServiceTime=0
  Timed to Evnt Signal : TimedToEventSignal
  Timed to Evnt Signal1 : TimedToEventSignal
  IN_Shipment_1 : PMIOPort  Port=1  Side=Left
  IN_Shipment_2 : PMIOPort  Port=2  Side=Left
  IN_Shipment_3 : PMIOPort  Port=3  Side=Left
  OUT_Shipment_1 : PMIOPort  Port=4  Side=Right
  OUT_Shipment_2 : PMIOPort  Port=5  Side=Right
  OUT_Shipment_3 : PMIOPort  Port=6  Side=Right
  wires:
  Timed to Evnt Signal1/1 -> MATLAB Function/3(lookup)
  Lookup/1 -> Timed to Evnt Signal1/1
  Timed to Evnt Signal/1 -> MATLAB Function/2(current)
  Get Attribute1/1 -> MATLAB Function/1(route)
  MATLAB Function/1(next) -> OUT_Shipment/1
  Node_ID/1 -> Timed to Evnt Signal/1
  Mux/1 -> Shipment_Metrics/1
  Get Attribute/3 -> Mux/3
  Get Attribute/2 -> Mux/2
  Get Attribute/1 -> Mux/1
  connections:
  Single Server/RConn1 -- OUT_Shipment/LConn1
  Get Attribute1/RConn1 -- Single Server/LConn1
  IN_Commodity/RConn1 -- Get Attribute1/LConn1
  Get Attribute/LConn1 -- IN_Shipment/RConn1
  Entity Sink/LConn1 -- Get Attribute/RConn1
  IN_Shipment/LConn1 -- IN_Shipment_1/RConn1
  IN_Shipment/LConn2 -- IN_Shipment_2/RConn1
  IN_Shipment/LConn3 -- IN_Shipment_3/RConn1
  OUT_Shipment/RConn1 -- OUT_Shipment_1/RConn1
  OUT_Shipment/RConn2 -- OUT_Shipment_2/RConn1
  OUT_Shipment/RConn3 -- OUT_Shipment_3/RConn1
  Commodity_26/RConn1 -- IN_Commodity/LConn1
  Commodity_27/RConn1 -- IN_Commodity/LConn2
  Commodity_28/RConn1 -- IN_Commodity/LConn3
  Commodity_29/RConn1 -- IN_Commodity/LConn4
  Commodity_30/RConn1 -- IN_Commodity/LConn5
  Commodity_31/RConn1 -- IN_Commodity/LConn6
  Commodity_32/RConn1 -- IN_Commodity/LConn7
  Commodity_33/RConn1 -- IN_Commodity/LConn8

== system Distribution_v2/Customer_5 ==
  Commodity_34 : Subsystem  mask{Mean=2000/427, AttributeValue=[5  22   1   0]|5|1|1}
      mask prompts: Mean "Frequency"; AttributeValue "Attributes"
  Commodity_35 : Subsystem  mask{Mean=2000/257, AttributeValue=[5  22  20   3]|5|3|1}
      mask prompts: Mean "Frequency"; AttributeValue "Attributes"
  Commodity_36 : Subsystem  mask{Mean=2000/38, AttributeValue=[5  22  18   4]|5|4|1}
      mask prompts: Mean "Frequency"; AttributeValue "Attributes"
  Commodity_37 : Subsystem  mask{Mean=2000/62, AttributeValue=[5  22  18   6]|5|6|1}
      mask prompts: Mean "Frequency"; AttributeValue "Attributes"
  Commodity_38 : Subsystem  mask{Mean=2000/120, AttributeValue=[5  22  20   7]|5|7|1}
      mask prompts: Mean "Frequency"; AttributeValue "Attributes"
  Commodity_39 : Subsystem  mask{Mean=2000/25, AttributeValue=[5  22  20   8]|5|8|1}
      mask prompts: Mean "Frequency"; AttributeValue "Attributes"
  Commodity_40 : Subsystem  mask{Mean=2000/245, AttributeValue=[5  22  20  11]|5|11|1}
      mask prompts: Mean "Frequency"; AttributeValue "Attributes"
  Commodity_41 : Subsystem  mask{Mean=2000/451, AttributeValue=[5  22  12   0]|5|12|1}
      mask prompts: Mean "Frequency"; AttributeValue "Attributes"
  Commodity_42 : Subsystem  mask{Mean=2000/56, AttributeValue=[5  22  13   0]|5|13|1}
      mask prompts: Mean "Frequency"; AttributeValue "Attributes"
  Commodity_43 : Subsystem  mask{Mean=2000/121, AttributeValue=[5  22  20  15]|5|15|1}
      mask prompts: Mean "Frequency"; AttributeValue "Attributes"
  Entity Sink : EntitySink
  Get Attribute : GetAttribute  AttributeName=Origin|Destination|Start  AttributeMissing=Error|Error|Error  AttributeDefaultValue=1|1|1  AttributeTreatAsVector=1|1|1  AttributeSendTiming=After entity departure|After entity departure|After entity departure  EvaluatedDefaultAttributeValue={[];[];[]}
      settings: OutputPortMap=o1,o2,o3
  Get Attribute1 : GetAttribute  AttributeName=Route  EvaluatedDefaultAttributeValue={[]}
      settings: OutputPortMap=o1
  IN_Commodity : PathCombiner  NumberInputPorts=10
  IN_Shipment : PathCombiner  NumberInputPorts=1
  Lookup : Constant  Value=[22]
  MATLAB Function : MATLAB Function  TreatAsAtomicUnit=on
  Mux : Mux  Inputs=3
  Node_ID : Constant  Value=5
  OUT_Shipment : OutputSwitch  NumberOutputPorts=1  SwitchingCriterion=From signal port p  AttributeName=Customer
  Shipment_Metrics : simeventslib/SimEvents Sinks/Discrete Event Signal to Workspace  VariableName=Customer_5  SaveFormat=Structure With Time  isMonitorOnly=off  isRecordIC=off
  Single Server : SingleServer  ServiceTime=0
  Timed to Evnt Signal : TimedToEventSignal
  Timed to Evnt Signal1 : TimedToEventSignal
  IN_Shipment_1 : PMIOPort  Port=1  Side=Left
  OUT_Shipment_1 : PMIOPort  Port=2  Side=Right
  wires:
  Timed to Evnt Signal1/1 -> MATLAB Function/3(lookup)
  Lookup/1 -> Timed to Evnt Signal1/1
  Timed to Evnt Signal/1 -> MATLAB Function/2(current)
  Get Attribute1/1 -> MATLAB Function/1(route)
  MATLAB Function/1(next) -> OUT_Shipment/1
  Node_ID/1 -> Timed to Evnt Signal/1
  Mux/1 -> Shipment_Metrics/1
  Get Attribute/3 -> Mux/3
  Get Attribute/2 -> Mux/2
  Get Attribute/1 -> Mux/1
  connections:
  Single Server/RConn1 -- OUT_Shipment/LConn1
  Get Attribute1/RConn1 -- Single Server/LConn1
  IN_Commodity/RConn1 -- Get Attribute1/LConn1
  Get Attribute/LConn1 -- IN_Shipment/RConn1
  Entity Sink/LConn1 -- Get Attribute/RConn1
  IN_Shipment/LConn1 -- IN_Shipment_1/RConn1
  OUT_Shipment/RConn1 -- OUT_Shipment_1/RConn1
  Commodity_34/RConn1 -- IN_Commodity/LConn1
  Commodity_35/RConn1 -- IN_Commodity/LConn2
  Commodity_36/RConn1 -- IN_Commodity/LConn3
  Commodity_37/RConn1 -- IN_Commodity/LConn4
  Commodity_38/RConn1 -- IN_Commodity/LConn5
  Commodity_39/RConn1 -- IN_Commodity/LConn6
  Commodity_40/RConn1 -- IN_Commodity/LConn7
  Commodity_41/RConn1 -- IN_Commodity/LConn8
  Commodity_42/RConn1 -- IN_Commodity/LConn9
  Commodity_43/RConn1 -- IN_Commodity/LConn10
